simulink model "ScriptDemo"  (R2022b)
settings: configuration reference "TmVcThermal_Configuration_sub" (kept outside this file)
undefined symbols (not defined in the file or in its folder): aaaa, bbbb, cTmComprCtrl_D_u8HvacFlowTable_db, cTmComprCtrl_D_u8HvacFlowTable_sw, cTmComprCtrl_n_i16ChillCmpIMax, cTmComprCtrl_n_i16ChillCmpIMin, cTmComprCtrl_n_i16ChillCmpIMin666, cTmComprCtrl_n_i16ChillCmpPMax, cTmComprCtrl_n_i16ChillCmpPMin, cTmComprCtrl_n_i16CmpChillCoolRpmKiMax, cTmComprCtrl_n_i16CmpChillCoolRpmKiMin, cTmComprCtrl_n_i16CmpChillCoolRpmKpMax, cTmComprCtrl_n_i16CmpChillCoolRpmKpMin, cTmComprCtrl_n_i16CmpCoolRpmKiMax, cTmComprCtrl_n_i16CmpCoolRpmKiMin, cTmComprCtrl_n_i16CmpCoolRpmKpMax, cTmComprCtrl_n_i16CmpCoolRpmKpMin, cTmComprCtrl_n_i16SM4CmpHeatKiMax, cTmComprCtrl_n_i16SM4CmpHeatKiMin, cTmComprCtrl_n_i16SM4CmpHeatKpMax, cTmComprCtrl_n_i16SM4CmpHeatKpMin, cTmComprCtrl_n_i16SM5CmpHeatKiMax, cTmComprCtrl_n_i16SM5CmpHeatKiMin, cTmComprCtrl_n_i16SM5CmpHeatKpMax, cTmComprCtrl_n_i16SM5CmpHeatKpMin, cTmComprCtrl_n_i16SM6CmpHeatKiMax, cTmComprCtrl_n_i16SM6CmpHeatKiMin, cTmComprCtrl_n_i16SM6CmpHeatKpMax, cTmComprCtrl_n_i16SM6CmpHeatKpMin, cTmComprCtrl_n_u16CmpMaxSpdFanFltLimt, cTmComprCtrl_n_u16CmpMaxSpdLoSidePFltLimt, cTmComprCtrl_n_u16CmpMaxSpdSensorFltLimt, cTmComprCtrl_n_u16CompMinRpm, cTmComprCtrl_n_u16CompRpmIncThres, cTmComprCtrl_t_u16BattCooltFFPeriod, cTmComprCtrl_t_u16BattCooltPIPeriod, cTmComprCtrl_t_u16CmpCoolFFPeriod, cTmComprCtrl_t_u16CmpCoolPIPeriod, cTmComprCtrl_t_u16CoolCmpChillFFPeriod, cTmComprCtrl_t_u16CoolCmpChillPIPeriod, cTmComprCtrl_t_u16SM4CmpHeatFFPeriod, cTmComprCtrl_t_u16SM4CmpHeatPIPeriod, cTmComprCtrl_t_u16SM5CmpHeatFFPeriod, cTmComprCtrl_t_u16SM5CmpHeatPIPeriod, cTmComprCtrl_t_u16SM6CmpHeatFFPeriod, cTmComprCtrl_t_u16SM6CmpHeatPIPeriod, cTmComprCtrl_Te_EvapClearInteg, cTmComprCtrl_Te_i16HpReqTempSaturoffset, cTmComprCtrl_Te_i16SatLpReplaceDiff, cTmComprCtrl_Te_i16SM3BatDiffStartEvapDecOffset, cTmComprCtrl_Te_i16SM3EvapLo, cTmComprCtrl_Te_i16SM3TBatDiffEntEvapDecOffset, cTmComprCtrl_Te_i16SM3TBatDiffEntEvapDecOffsetQuit, cTmComprCtrl_Te_s32ErrCmpChillPIContinueCoolH, cTmComprCtrl_Te_s32ErrCmpChillPIContinueCoolL, cTmComprCtrl_Te_s32ErrCmpPIContinueChillH, cTmComprCtrl_Te_s32ErrCmpPIContinueChillL, cTmComprCtrl_Te_s32ErrCmpPIContinueCoolH, cTmComprCtrl_Te_s32ErrCmpPIContinueCoolL, cTmComprCtrl_Te_s32ErrCmpPIContinueHeatH ... (+398)
libraries: simulink x846, PCMULib x711, simulink_need_slupdate x4
(part 47 of 49)

== system ScriptDemo/Create/createMerge/After/SM3SM23/ID26262_SM3FF/SM3SM2FF/Flow2RpmRec1/Subsystem5 ==
  In1 : Inport  OutDataTypeStr=int16
  Abs : Abs  OutDataTypeStr=uint16  SaturateOnIntegerOverflow=off
  Add6 : Sum  Inputs=+-  OutDataTypeStr=int16
  Compare To Constant : simulink/Logic and Bit Operations/Compare To Constant  relop=>=  const=0  OutDataTypeStr=boolean
  Compare To Constant1 : simulink/Logic and Bit Operations/Compare To Constant  relop=<=  const=10  OutDataTypeStr=boolean
  Constant6 : Constant  Value=0  OutDataTypeStr=uint16
  Constant7 : Constant  Value=10  OutDataTypeStr=uint16
  Logical Operator : Logic  AllPortsSameDT=off  OutDataTypeStr=boolean
  Switch : Switch  Criteria=u2 ~= 0  SaturateOnIntegerOverflow=off  InputSameDT=off
  Out1 : Outport
  wires:
  Add6/1 -> Switch/1
  Logical Operator/1 -> Switch/2
  Constant6/1 -> Switch/3
  Abs/1 -> Add6/2, Compare To Constant/1, Compare To Constant1/1
  Constant7/1 -> Add6/1
  Switch/1 -> Out1/1
  Compare To Constant1/1 -> Logical Operator/2
  Compare To Constant/1 -> Logical Operator/1
  In1/1 -> Abs/1

== system ScriptDemo/Create/createMerge/After/SM3SM23/ID26262_SM3FF/SM3SM2FF/Flow2RpmRec1/XCP ==
  md_u8Blw : Inport
  Constant1 : Constant  Value=BlwHeatLevel_db
      settings: AttributesFormatString=%<Value>
  Constant28 : Constant  Value=BlwHeatLevel_sw
      settings: AttributesFormatString=%<Value>
  Switch : Switch  Criteria=u2 ~= 0  SaturateOnIntegerOverflow=off  InputSameDT=off
  Out1 : Outport
  wires:
  md_u8Blw/1 -> Switch/3
  Switch/1 -> Out1/1
  Constant28/1 -> Switch/2
  Constant1/1 -> Switch/1

== system ScriptDemo/Create/createMerge/After/SM3SM23/ID26263_SM3Error/SM3HPErr/isNeedOffset/Timer Running2 ==
  note: CounterRunning
  note: If timer is set to zero, use start/hold/reset-status as output.
      | This is to avoid TimerFinished to be set to true without even the timer has started.
  Start : Inport  OutDataTypeStr=boolean
  Reset : Inport  Port=2  OutDataTypeStr=boolean
  Time : Inport  Port=3  OutDataTypeStr=uint16
  Divide : Product  Inputs=*/  OutDataTypeStr=uint32  RndMeth=Round  SaturateOnIntegerOverflow=on
  IC : Constant  Value=0  OutDataTypeStr=uint32  SampleTime=-1
  Increment : Constant  OutDataTypeStr=uint32  SampleTime=-1
  Logical Operator : Logic  AllPortsSameDT=off  OutDataTypeStr=boolean
  Logical Operator2 : Logic  Operator=OR  AllPortsSameDT=off  OutDataTypeStr=boolean
  Logical Operator3 : Logic  Operator=NOT  AllPortsSameDT=off  OutDataTypeStr=boolean
  Relational Operator : RelationalOperator  OutDataTypeStr=boolean  InputSameDT=off
  Relational Operator1 : RelationalOperator  Operator=>  OutDataTypeStr=boolean  InputSameDT=off
  RunnablePeriod : Constant  Value=cTmSwArch_t_s32SampleTime  OutDataTypeStr=single  SampleTime=-1
  StopCounter : Constant  Value=0  OutDataTypeStr=uint32  SampleTime=-1
  Sum : Sum  OutDataTypeStr=uint32  SaturateOnIntegerOverflow=on
  Switch : Switch  Criteria=u2 ~= 0  InputSameDT=off
  Switch1 : Switch  Criteria=u2 ~= 0  InputSameDT=off
  Unit Delay External IC : simulink_need_slupdate/Unit Delay External IC  tsamp=-1
  Unit Delay Resettable External IC1 : Subsystem  AncestorBlock=|  mask(Unit Delay Resettable External Initial Condition NGCC v1.0){dataType=uint32}
      | CCMLib/Unit Delay
      | Resettable
      | External IC
      mask prompts: dataType "Data type:"
      mask help:
      | NGCC version of the Simulink built-in block with data type control and boolean datatype usage for internal switch condition.
      | -----------------------------------------------------
      | Normally, the output is the signal u delayed by one sample period.
      | When the reset signal R is true, the state and the output are always set equal to the initial condition signal IC.  This reset action is vectorized and supports scalar expansion.
      |
      | Mx-VDev tested: Yes
      mask TypeOptions dataType: uint8 | uint16 | uint32 | single
      mask Display: dpoly(1,[1 0],'z')
  ZeroTicks : Constant  Value=0  OutDataTypeStr=uint32  SampleTime=-1
  false : Constant  Value=false  OutDataTypeStr=boolean  SampleTime=-1
  TimerFinished : Outport  OutDataTypeStr=boolean
  TimerRunning : Outport  Port=2  OutDataTypeStr=boolean
  wires:
  Logical Operator2/1 -> Logical Operator/1
  false/1 -> Unit Delay External IC/2
  Logical Operator/1 -> Switch/2, Unit Delay External IC/1, Switch1/3, TimerRunning/1
  Start/1 -> Logical Operator2/2
  Unit Delay External IC/1 -> Logical Operator2/1
  Unit Delay Resettable External IC1/1(y) -> Relational Operator/1, Sum/1
  Switch/1 -> Sum/2
  Increment/1 -> Switch/1
  StopCounter/1 -> Switch/3
  RunnablePeriod/1 -> Divide/2
  ZeroTicks/1 -> Relational Operator1/2
  Relational Operator1/1 -> Switch1/2
  Relational Operator/1 -> Switch1/1
  Divide/1 -> Relational Operator/2, Relational Operator1/1
  Switch1/1 -> TimerFinished/1
  Logical Operator3/1 -> Logical Operator/2
  Reset/1 -> Logical Operator3/1, Unit Delay Resettable External IC1/3(R)
  Time/1 -> Divide/1
  IC/1 -> Unit Delay Resettable External IC1/2(IC)
  Sum/1 -> Unit Delay Resettable External IC1/1(u)

== system ScriptDemo/Create/createMerge/After/SM3SM23/SM3_Ki/SM2Ki/Flow2Rpm/Subsystem1 ==
  In1 : Inport  OutDataTypeStr=int16
  Abs : Abs  OutDataTypeStr=single  SaturateOnIntegerOverflow=off
  Add6 : Sum  Inputs=+-  OutDataTypeStr=int16
  Compare To Constant : simulink/Logic and Bit Operations/Compare To Constant  relop=>=  const=0  OutDataTypeStr=boolean
  Compare To Constant1 : simulink/Logic and Bit Operations/Compare To Constant  relop=<=  const=10  OutDataTypeStr=boolean
  Constant6 : Constant  Value=0  OutDataTypeStr=uint16
  Constant7 : Constant  Value=10  OutDataTypeStr=uint16
  Logical Operator : Logic  AllPortsSameDT=off  OutDataTypeStr=boolean
  Switch : Switch  Criteria=u2 ~= 0  SaturateOnIntegerOverflow=off  InputSameDT=off
  Out1 : Outport
  wires:
  Add6/1 -> Switch/1
  Logical Operator/1 -> Switch/2
  Constant6/1 -> Switch/3
  Abs/1 -> Add6/2, Compare To Constant/1, Compare To Constant1/1
  Constant7/1 -> Add6/1
  Switch/1 -> Out1/1
  Compare To Constant1/1 -> Logical Operator/2
  Compare To Constant/1 -> Logical Operator/1
  In1/1 -> Abs/1

== system ScriptDemo/Create/createMerge/After/SM3SM23/SM3_Ki/SM2Ki/Flow2Rpm/Subsystem2 ==
  In1 : Inport  OutDataTypeStr=int16
  Abs : Abs  OutDataTypeStr=uint16  SaturateOnIntegerOverflow=off
  Add6 : Sum  Inputs=+-  OutDataTypeStr=int16
  Compare To Constant : simulink/Logic and Bit Operations/Compare To Constant  relop=>=  const=0  OutDataTypeStr=boolean
  Compare To Constant1 : simulink/Logic and Bit Operations/Compare To Constant  relop=<=  const=10  OutDataTypeStr=boolean
  Constant6 : Constant  Value=0  OutDataTypeStr=uint16
  Constant7 : Constant  Value=10  OutDataTypeStr=uint16
  Logical Operator : Logic  AllPortsSameDT=off  OutDataTypeStr=boolean
  Switch : Switch  Criteria=u2 ~= 0  SaturateOnIntegerOverflow=off  InputSameDT=off
  Out1 : Outport
  wires:
  Add6/1 -> Switch/1
  Logical Operator/1 -> Switch/2
  Constant6/1 -> Switch/3
  Abs/1 -> Add6/2, Compare To Constant/1, Compare To Constant1/1
  Constant7/1 -> Add6/1
  Switch/1 -> Out1/1
  Compare To Constant1/1 -> Logical Operator/2
  Compare To Constant/1 -> Logical Operator/1
  In1/1 -> Abs/1

== system ScriptDemo/Create/createMerge/After/SM3SM23/SM3_Ki/SM2Ki/Flow2Rpm/Subsystem3 ==
  In1 : Inport  OutDataTypeStr=int16
  Abs : Abs  OutDataTypeStr=uint16  SaturateOnIntegerOverflow=off
  Add6 : Sum  Inputs=+-  OutDataTypeStr=int16
  Compare To Constant : simulink/Logic and Bit Operations/Compare To Constant  relop=>=  const=0  OutDataTypeStr=boolean
  Compare To Constant1 : simulink/Logic and Bit Operations/Compare To Constant  relop=<=  const=10  OutDataTypeStr=boolean
  Constant6 : Constant  Value=0  OutDataTypeStr=uint16
  Constant7 : Constant  Value=10  OutDataTypeStr=uint16
  Logical Operator : Logic  AllPortsSameDT=off  OutDataTypeStr=boolean
  Switch : Switch  Criteria=u2 ~= 0  SaturateOnIntegerOverflow=off  InputSameDT=off
  Out1 : Outport
  wires:
  Add6/1 -> Switch/1
  Logical Operator/1 -> Switch/2
  Constant6/1 -> Switch/3
  Abs/1 -> Add6/2, Compare To Constant/1, Compare To Constant1/1
  Constant7/1 -> Add6/1
  Switch/1 -> Out1/1
  Compare To Constant1/1 -> Logical Operator/2
  Compare To Constant/1 -> Logical Operator/1
  In1/1 -> Abs/1

== system ScriptDemo/Create/createMerge/After/SM3SM23/SM3_Ki/SM2Ki/Flow2Rpm/Subsystem4 ==
  In1 : Inport  OutDataTypeStr=int16
  Abs : Abs  OutDataTypeStr=uint16  SaturateOnIntegerOverflow=off
  Add6 : Sum  Inputs=+-  OutDataTypeStr=int16
  Compare To Constant : simulink/Logic and Bit Operations/Compare To Constant  relop=>=  const=0  OutDataTypeStr=boolean
  Compare To Constant1 : simulink/Logic and Bit Operations/Compare To Constant  relop=<=  const=10  OutDataTypeStr=boolean
  Constant6 : Constant  Value=0  OutDataTypeStr=uint16
  Constant7 : Constant  Value=10  OutDataTypeStr=uint16
  Logical Operator : Logic  AllPortsSameDT=off  OutDataTypeStr=boolean
  Switch : Switch  Criteria=u2 ~= 0  SaturateOnIntegerOverflow=off  InputSameDT=off
  Out1 : Outport
  wires:
  Add6/1 -> Switch/1
  Logical Operator/1 -> Switch/2
  Constant6/1 -> Switch/3
  Abs/1 -> Add6/2, Compare To Constant/1, Compare To Constant1/1
  Constant7/1 -> Add6/1
  Switch/1 -> Out1/1
  Compare To Constant1/1 -> Logical Operator/2
  Compare To Constant/1 -> Logical Operator/1
  In1/1 -> Abs/1

== system ScriptDemo/Create/createMerge/After/SM3SM23/SM3_Ki/SM2Ki/Flow2Rpm/Subsystem5 ==
  In1 : Inport  OutDataTypeStr=int16
  Abs : Abs  OutDataTypeStr=uint16  SaturateOnIntegerOverflow=off
  Add6 : Sum  Inputs=+-  OutDataTypeStr=int16
  Compare To Constant : simulink/Logic and Bit Operations/Compare To Constant  relop=>=  const=0  OutDataTypeStr=boolean
  Compare To Constant1 : simulink/Logic and Bit Operations/Compare To Constant  relop=<=  const=10  OutDataTypeStr=boolean
  Constant6 : Constant  Value=0  OutDataTypeStr=uint16
  Constant7 : Constant  Value=10  OutDataTypeStr=uint16
  Logical Operator : Logic  AllPortsSameDT=off  OutDataTypeStr=boolean
  Switch : Switch  Criteria=u2 ~= 0  SaturateOnIntegerOverflow=off  InputSameDT=off
  Out1 : Outport
  wires:
  Add6/1 -> Switch/1
  Logical Operator/1 -> Switch/2
  Constant6/1 -> Switch/3
  Abs/1 -> Add6/2, Compare To Constant/1, Compare To Constant1/1
  Constant7/1 -> Add6/1
  Switch/1 -> Out1/1
  Compare To Constant1/1 -> Logical Operator/2
  Compare To Constant/1 -> Logical Operator/1
  In1/1 -> Abs/1

== system ScriptDemo/Create/createMerge/After/SM3SM23/SM3_Ki/SM2Ki/Flow2Rpm/XCP ==
  md_u8Blw : Inport
  Constant1 : Constant  Value=BlwHeatLevel_db
      settings: AttributesFormatString=%<Value>
  Constant28 : Constant  Value=BlwHeatLevel_sw
      settings: AttributesFormatString=%<Value>
  Switch : Switch  Criteria=u2 ~= 0  SaturateOnIntegerOverflow=off  InputSameDT=off
  Out1 : Outport
  wires:
  md_u8Blw/1 -> Switch/3
  Switch/1 -> Out1/1
  Constant28/1 -> Switch/2
  Constant1/1 -> Switch/1

== system ScriptDemo/Create/createMerge/After/SM3SM23/SM3_Ki/SM2Ki/Flow2Rpm1/Subsystem1 ==
  In1 : Inport  OutDataTypeStr=int16
  Abs : Abs  OutDataTypeStr=single  SaturateOnIntegerOverflow=off
  Add6 : Sum  Inputs=+-  OutDataTypeStr=int16
  Compare To Constant : simulink/Logic and Bit Operations/Compare To Constant  relop=>=  const=0  OutDataTypeStr=boolean
  Compare To Constant1 : simulink/Logic and Bit Operations/Compare To Constant  relop=<=  const=10  OutDataTypeStr=boolean
  Constant6 : Constant  Value=0  OutDataTypeStr=uint16
  Constant7 : Constant  Value=10  OutDataTypeStr=uint16
  Logical Operator : Logic  AllPortsSameDT=off  OutDataTypeStr=boolean
  Switch : Switch  Criteria=u2 ~= 0  SaturateOnIntegerOverflow=off  InputSameDT=off
  Out1 : Outport
  wires:
  Add6/1 -> Switch/1
  Logical Operator/1 -> Switch/2
  Constant6/1 -> Switch/3
  Abs/1 -> Add6/2, Compare To Constant/1, Compare To Constant1/1
  Constant7/1 -> Add6/1
  Switch/1 -> Out1/1
  Compare To Constant1/1 -> Logical Operator/2
  Compare To Constant/1 -> Logical Operator/1
  In1/1 -> Abs/1

== system ScriptDemo/Create/createMerge/After/SM3SM23/SM3_Ki/SM2Ki/Flow2Rpm1/Subsystem2 ==
  In1 : Inport  OutDataTypeStr=int16
  Abs : Abs  OutDataTypeStr=uint16  SaturateOnIntegerOverflow=off
  Add6 : Sum  Inputs=+-  OutDataTypeStr=int16
  Compare To Constant : simulink/Logic and Bit Operations/Compare To Constant  relop=>=  const=0  OutDataTypeStr=boolean
  Compare To Constant1 : simulink/Logic and Bit Operations/Compare To Constant  relop=<=  const=10  OutDataTypeStr=boolean
  Constant6 : Constant  Value=0  OutDataTypeStr=uint16
  Constant7 : Constant  Value=10  OutDataTypeStr=uint16
  Logical Operator : Logic  AllPortsSameDT=off  OutDataTypeStr=boolean
  Switch : Switch  Criteria=u2 ~= 0  SaturateOnIntegerOverflow=off  InputSameDT=off
  Out1 : Outport
  wires:
  Add6/1 -> Switch/1
  Logical Operator/1 -> Switch/2
  Constant6/1 -> Switch/3
  Abs/1 -> Add6/2, Compare To Constant/1, Compare To Constant1/1
  Constant7/1 -> Add6/1
  Switch/1 -> Out1/1
  Compare To Constant1/1 -> Logical Operator/2
  Compare To Constant/1 -> Logical Operator/1
  In1/1 -> Abs/1

== system ScriptDemo/Create/createMerge/After/SM3SM23/SM3_Ki/SM2Ki/Flow2Rpm1/Subsystem3 ==
  In1 : Inport  OutDataTypeStr=int16
  Abs : Abs  OutDataTypeStr=uint16  SaturateOnIntegerOverflow=off
  Add6 : Sum  Inputs=+-  OutDataTypeStr=int16
  Compare To Constant : simulink/Logic and Bit Operations/Compare To Constant  relop=>=  const=0  OutDataTypeStr=boolean
  Compare To Constant1 : simulink/Logic and Bit Operations/Compare To Constant  relop=<=  const=10  OutDataTypeStr=boolean
  Constant6 : Constant  Value=0  OutDataTypeStr=uint16
  Constant7 : Constant  Value=10  OutDataTypeStr=uint16
  Logical Operator : Logic  AllPortsSameDT=off  OutDataTypeStr=boolean
  Switch : Switch  Criteria=u2 ~= 0  SaturateOnIntegerOverflow=off  InputSameDT=off
  Out1 : Outport
  wires:
  Add6/1 -> Switch/1
  Logical Operator/1 -> Switch/2
  Constant6/1 -> Switch/3
  Abs/1 -> Add6/2, Compare To Constant/1, Compare To Constant1/1
  Constant7/1 -> Add6/1
  Switch/1 -> Out1/1
  Compare To Constant1/1 -> Logical Operator/2
  Compare To Constant/1 -> Logical Operator/1
  In1/1 -> Abs/1

== system ScriptDemo/Create/createMerge/After/SM3SM23/SM3_Ki/SM2Ki/Flow2Rpm1/Subsystem4 ==
  In1 : Inport  OutDataTypeStr=int16
  Abs : Abs  OutDataTypeStr=uint16  SaturateOnIntegerOverflow=off
  Add6 : Sum  Inputs=+-  OutDataTypeStr=int16
  Compare To Constant : simulink/Logic and Bit Operations/Compare To Constant  relop=>=  const=0  OutDataTypeStr=boolean
  Compare To Constant1 : simulink/Logic and Bit Operations/Compare To Constant  relop=<=  const=10  OutDataTypeStr=boolean
  Constant6 : Constant  Value=0  OutDataTypeStr=uint16
  Constant7 : Constant  Value=10  OutDataTypeStr=uint16
  Logical Operator : Logic  AllPortsSameDT=off  OutDataTypeStr=boolean
  Switch : Switch  Criteria=u2 ~= 0  SaturateOnIntegerOverflow=off  InputSameDT=off
  Out1 : Outport
  wires:
  Add6/1 -> Switch/1
  Logical Operator/1 -> Switch/2
  Constant6/1 -> Switch/3
  Abs/1 -> Add6/2, Compare To Constant/1, Compare To Constant1/1
  Constant7/1 -> Add6/1
  Switch/1 -> Out1/1
  Compare To Constant1/1 -> Logical Operator/2
  Compare To Constant/1 -> Logical Operator/1
  In1/1 -> Abs/1

== system ScriptDemo/Create/createMerge/After/SM3SM23/SM3_Ki/SM2Ki/Flow2Rpm1/Subsystem5 ==
  In1 : Inport  OutDataTypeStr=int16
  Abs : Abs  OutDataTypeStr=uint16  SaturateOnIntegerOverflow=off
  Add6 : Sum  Inputs=+-  OutDataTypeStr=int16
  Compare To Constant : simulink/Logic and Bit Operations/Compare To Constant  relop=>=  const=0  OutDataTypeStr=boolean
  Compare To Constant1 : simulink/Logic and Bit Operations/Compare To Constant  relop=<=  const=10  OutDataTypeStr=boolean
  Constant6 : Constant  Value=0  OutDataTypeStr=uint16
  Constant7 : Constant  Value=10  OutDataTypeStr=uint16
  Logical Operator : Logic  AllPortsSameDT=off  OutDataTypeStr=boolean
  Switch : Switch  Criteria=u2 ~= 0  SaturateOnIntegerOverflow=off  InputSameDT=off
  Out1 : Outport
  wires:
  Add6/1 -> Switch/1
  Logical Operator/1 -> Switch/2
  Constant6/1 -> Switch/3
  Abs/1 -> Add6/2, Compare To Constant/1, Compare To Constant1/1
  Constant7/1 -> Add6/1
  Switch/1 -> Out1/1
  Compare To Constant1/1 -> Logical Operator/2
  Compare To Constant/1 -> Logical Operator/1
  In1/1 -> Abs/1

== system ScriptDemo/Create/createMerge/After/SM3SM23/SM3_Ki/SM2Ki/Flow2Rpm1/XCP ==
  md_u8Blw : Inport
  Constant1 : Constant  Value=BlwHeatLevel_db
      settings: AttributesFormatString=%<Value>
  Constant28 : Constant  Value=BlwHeatLevel_sw
      settings: AttributesFormatString=%<Value>
  Switch : Switch  Criteria=u2 ~= 0  SaturateOnIntegerOverflow=off  InputSameDT=off
  Out1 : Outport
  wires:
  md_u8Blw/1 -> Switch/3
  Switch/1 -> Out1/1
  Constant28/1 -> Switch/2
  Constant1/1 -> Switch/1

== system ScriptDemo/Create/createMerge/After/SM3SM23/SM3_Ki/SM3SM2LikeKi/Osa/Subsystem1 ==
  In1 : Inport  OutDataTypeStr=int16
  Abs : Abs  OutDataTypeStr=single  SaturateOnIntegerOverflow=off
  Add6 : Sum  Inputs=+-  OutDataTypeStr=int16
  Compare To Constant : simulink/Logic and Bit Operations/Compare To Constant  relop=>=  const=0  OutDataTypeStr=boolean
  Compare To Constant1 : simulink/Logic and Bit Operations/Compare To Constant  relop=<=  const=10  OutDataTypeStr=boolean
  Constant6 : Constant  Value=0  OutDataTypeStr=uint16
  Constant7 : Constant  Value=10  OutDataTypeStr=uint16
  Logical Operator : Logic  AllPortsSameDT=off  OutDataTypeStr=boolean
  Switch : Switch  Criteria=u2 ~= 0  SaturateOnIntegerOverflow=off  InputSameDT=off
  Out1 : Outport
  wires:
  Add6/1 -> Switch/1
  Logical Operator/1 -> Switch/2
  Constant6/1 -> Switch/3
  Abs/1 -> Add6/2, Compare To Constant/1, Compare To Constant1/1
  Constant7/1 -> Add6/1
  Switch/1 -> Out1/1
  Compare To Constant1/1 -> Logical Operator/2
  Compare To Constant/1 -> Logical Operator/1
  In1/1 -> Abs/1

== system ScriptDemo/Create/createMerge/After/SM3SM23/SM3_Ki/SM3SM2LikeKi/Osa/Subsystem2 ==
  In1 : Inport  OutDataTypeStr=int16
  Abs : Abs  OutDataTypeStr=uint16  SaturateOnIntegerOverflow=off
  Add6 : Sum  Inputs=+-  OutDataTypeStr=int16
  Compare To Constant : simulink/Logic and Bit Operations/Compare To Constant  relop=>=  const=0  OutDataTypeStr=boolean
  Compare To Constant1 : simulink/Logic and Bit Operations/Compare To Constant  relop=<=  const=10  OutDataTypeStr=boolean
  Constant6 : Constant  Value=0  OutDataTypeStr=uint16
  Constant7 : Constant  Value=10  OutDataTypeStr=uint16
  Logical Operator : Logic  AllPortsSameDT=off  OutDataTypeStr=boolean
  Switch : Switch  Criteria=u2 ~= 0  SaturateOnIntegerOverflow=off  InputSameDT=off
  Out1 : Outport
  wires:
  Add6/1 -> Switch/1
  Logical Operator/1 -> Switch/2
  Constant6/1 -> Switch/3
  Abs/1 -> Add6/2, Compare To Constant/1, Compare To Constant1/1
  Constant7/1 -> Add6/1
  Switch/1 -> Out1/1
  Compare To Constant1/1 -> Logical Operator/2
  Compare To Constant/1 -> Logical Operator/1
  In1/1 -> Abs/1

== system ScriptDemo/Create/createMerge/After/SM3SM23/SM3_Ki/SM3SM2LikeKi/Osa/Subsystem3 ==
  In1 : Inport  OutDataTypeStr=int16
  Abs : Abs  OutDataTypeStr=uint16  SaturateOnIntegerOverflow=off
  Add6 : Sum  Inputs=+-  OutDataTypeStr=int16
  Compare To Constant : simulink/Logic and Bit Operations/Compare To Constant  relop=>=  const=0  OutDataTypeStr=boolean
  Compare To Constant1 : simulink/Logic and Bit Operations/Compare To Constant  relop=<=  const=10  OutDataTypeStr=boolean
  Constant6 : Constant  Value=0  OutDataTypeStr=uint16
  Constant7 : Constant  Value=10  OutDataTypeStr=uint16
  Logical Operator : Logic  AllPortsSameDT=off  OutDataTypeStr=boolean
  Switch : Switch  Criteria=u2 ~= 0  SaturateOnIntegerOverflow=off  InputSameDT=off
  Out1 : Outport
  wires:
  Add6/1 -> Switch/1
  Logical Operator/1 -> Switch/2
  Constant6/1 -> Switch/3
  Abs/1 -> Add6/2, Compare To Constant/1, Compare To Constant1/1
  Constant7/1 -> Add6/1
  Switch/1 -> Out1/1
  Compare To Constant1/1 -> Logical Operator/2
  Compare To Constant/1 -> Logical Operator/1
  In1/1 -> Abs/1

== system ScriptDemo/Create/createMerge/After/SM3SM23/SM3_Ki/SM3SM2LikeKi/Osa/Subsystem4 ==
  In1 : Inport  OutDataTypeStr=int16
  Abs : Abs  OutDataTypeStr=uint16  SaturateOnIntegerOverflow=off
  Add6 : Sum  Inputs=+-  OutDataTypeStr=int16
  Compare To Constant : simulink/Logic and Bit Operations/Compare To Constant  relop=>=  const=0  OutDataTypeStr=boolean
  Compare To Constant1 : simulink/Logic and Bit Operations/Compare To Constant  relop=<=  const=10  OutDataTypeStr=boolean
  Constant6 : Constant  Value=0  OutDataTypeStr=uint16
  Constant7 : Constant  Value=10  OutDataTypeStr=uint16
  Logical Operator : Logic  AllPortsSameDT=off  OutDataTypeStr=boolean
  Switch : Switch  Criteria=u2 ~= 0  SaturateOnIntegerOverflow=off  InputSameDT=off
  Out1 : Outport
  wires:
  Add6/1 -> Switch/1
  Logical Operator/1 -> Switch/2
  Constant6/1 -> Switch/3
  Abs/1 -> Add6/2, Compare To Constant/1, Compare To Constant1/1
  Constant7/1 -> Add6/1
  Switch/1 -> Out1/1
  Compare To Constant1/1 -> Logical Operator/2
  Compare To Constant/1 -> Logical Operator/1
  In1/1 -> Abs/1

== system ScriptDemo/Create/createMerge/After/SM3SM23/SM3_Ki/SM3SM2LikeKi/Osa/Subsystem5 ==
  In1 : Inport  OutDataTypeStr=int16
  Abs : Abs  OutDataTypeStr=uint16  SaturateOnIntegerOverflow=off
  Add6 : Sum  Inputs=+-  OutDataTypeStr=int16
  Compare To Constant : simulink/Logic and Bit Operations/Compare To Constant  relop=>=  const=0  OutDataTypeStr=boolean
  Compare To Constant1 : simulink/Logic and Bit Operations/Compare To Constant  relop=<=  const=10  OutDataTypeStr=boolean
  Constant6 : Constant  Value=0  OutDataTypeStr=uint16
  Constant7 : Constant  Value=10  OutDataTypeStr=uint16
  Logical Operator : Logic  AllPortsSameDT=off  OutDataTypeStr=boolean
  Switch : Switch  Criteria=u2 ~= 0  SaturateOnIntegerOverflow=off  InputSameDT=off
  Out1 : Outport
  wires:
  Add6/1 -> Switch/1
  Logical Operator/1 -> Switch/2
  Constant6/1 -> Switch/3
  Abs/1 -> Add6/2, Compare To Constant/1, Compare To Constant1/1
  Constant7/1 -> Add6/1
  Switch/1 -> Out1/1
  Compare To Constant1/1 -> Logical Operator/2
  Compare To Constant/1 -> Logical Operator/1
  In1/1 -> Abs/1

== system ScriptDemo/Create/createMerge/After/SM3SM23/SM3_Ki/SM3SM2LikeKi/Osa/XCP ==
  md_u8Blw : Inport
  Constant1 : Constant  Value=BlwHeatLevel_db
      settings: AttributesFormatString=%<Value>
  Constant28 : Constant  Value=BlwHeatLevel_sw
      settings: AttributesFormatString=%<Value>
  Switch : Switch  Criteria=u2 ~= 0  SaturateOnIntegerOverflow=off  InputSameDT=off
  Out1 : Outport
  wires:
  md_u8Blw/1 -> Switch/3
  Switch/1 -> Out1/1
  Constant28/1 -> Switch/2
  Constant1/1 -> Switch/1

== system ScriptDemo/Create/createMerge/After/SM3SM23/SM3_Ki/SM3SM2LikeKi/Rec/Subsystem1 ==
  In1 : Inport  OutDataTypeStr=int16
  Abs : Abs  OutDataTypeStr=single  SaturateOnIntegerOverflow=off
  Add6 : Sum  Inputs=+-  OutDataTypeStr=int16
  Compare To Constant : simulink/Logic and Bit Operations/Compare To Constant  relop=>=  const=0  OutDataTypeStr=boolean
  Compare To Constant1 : simulink/Logic and Bit Operations/Compare To Constant  relop=<=  const=10  OutDataTypeStr=boolean
  Constant6 : Constant  Value=0  OutDataTypeStr=uint16
  Constant7 : Constant  Value=10  OutDataTypeStr=uint16
  Logical Operator : Logic  AllPortsSameDT=off  OutDataTypeStr=boolean
  Switch : Switch  Criteria=u2 ~= 0  SaturateOnIntegerOverflow=off  InputSameDT=off
  Out1 : Outport
  wires:
  Add6/1 -> Switch/1
  Logical Operator/1 -> Switch/2
  Constant6/1 -> Switch/3
  Abs/1 -> Add6/2, Compare To Constant/1, Compare To Constant1/1
  Constant7/1 -> Add6/1
  Switch/1 -> Out1/1
  Compare To Constant1/1 -> Logical Operator/2
  Compare To Constant/1 -> Logical Operator/1
  In1/1 -> Abs/1

== system ScriptDemo/Create/createMerge/After/SM3SM23/SM3_Ki/SM3SM2LikeKi/Rec/Subsystem2 ==
  In1 : Inport  OutDataTypeStr=int16
  Abs : Abs  OutDataTypeStr=uint16  SaturateOnIntegerOverflow=off
  Add6 : Sum  Inputs=+-  OutDataTypeStr=int16
  Compare To Constant : simulink/Logic and Bit Operations/Compare To Constant  relop=>=  const=0  OutDataTypeStr=boolean
  Compare To Constant1 : simulink/Logic and Bit Operations/Compare To Constant  relop=<=  const=10  OutDataTypeStr=boolean
  Constant6 : Constant  Value=0  OutDataTypeStr=uint16
  Constant7 : Constant  Value=10  OutDataTypeStr=uint16
  Logical Operator : Logic  AllPortsSameDT=off  OutDataTypeStr=boolean
  Switch : Switch  Criteria=u2 ~= 0  SaturateOnIntegerOverflow=off  InputSameDT=off
  Out1 : Outport
  wires:
  Add6/1 -> Switch/1
  Logical Operator/1 -> Switch/2
  Constant6/1 -> Switch/3
  Abs/1 -> Add6/2, Compare To Constant/1, Compare To Constant1/1
  Constant7/1 -> Add6/1
  Switch/1 -> Out1/1
  Compare To Constant1/1 -> Logical Operator/2
  Compare To Constant/1 -> Logical Operator/1
  In1/1 -> Abs/1

== system ScriptDemo/Create/createMerge/After/SM3SM23/SM3_Ki/SM3SM2LikeKi/Rec/Subsystem3 ==
  In1 : Inport  OutDataTypeStr=int16
  Abs : Abs  OutDataTypeStr=uint16  SaturateOnIntegerOverflow=off
  Add6 : Sum  Inputs=+-  OutDataTypeStr=int16
  Compare To Constant : simulink/Logic and Bit Operations/Compare To Constant  relop=>=  const=0  OutDataTypeStr=boolean
  Compare To Constant1 : simulink/Logic and Bit Operations/Compare To Constant  relop=<=  const=10  OutDataTypeStr=boolean
  Constant6 : Constant  Value=0  OutDataTypeStr=uint16
  Constant7 : Constant  Value=10  OutDataTypeStr=uint16
  Logical Operator : Logic  AllPortsSameDT=off  OutDataTypeStr=boolean
  Switch : Switch  Criteria=u2 ~= 0  SaturateOnIntegerOverflow=off  InputSameDT=off
  Out1 : Outport
  wires:
  Add6/1 -> Switch/1
  Logical Operator/1 -> Switch/2
  Constant6/1 -> Switch/3
  Abs/1 -> Add6/2, Compare To Constant/1, Compare To Constant1/1
  Constant7/1 -> Add6/1
  Switch/1 -> Out1/1
  Compare To Constant1/1 -> Logical Operator/2
  Compare To Constant/1 -> Logical Operator/1
  In1/1 -> Abs/1

== system ScriptDemo/Create/createMerge/After/SM3SM23/SM3_Ki/SM3SM2LikeKi/Rec/Subsystem4 ==
  In1 : Inport  OutDataTypeStr=int16
  Abs : Abs  OutDataTypeStr=uint16  SaturateOnIntegerOverflow=off
  Add6 : Sum  Inputs=+-  OutDataTypeStr=int16
  Compare To Constant : simulink/Logic and Bit Operations/Compare To Constant  relop=>=  const=0  OutDataTypeStr=boolean
  Compare To Constant1 : simulink/Logic and Bit Operations/Compare To Constant  relop=<=  const=10  OutDataTypeStr=boolean
  Constant6 : Constant  Value=0  OutDataTypeStr=uint16
  Constant7 : Constant  Value=10  OutDataTypeStr=uint16
  Logical Operator : Logic  AllPortsSameDT=off  OutDataTypeStr=boolean
  Switch : Switch  Criteria=u2 ~= 0  SaturateOnIntegerOverflow=off  InputSameDT=off
  Out1 : Outport
  wires:
  Add6/1 -> Switch/1
  Logical Operator/1 -> Switch/2
  Constant6/1 -> Switch/3
  Abs/1 -> Add6/2, Compare To Constant/1, Compare To Constant1/1
  Constant7/1 -> Add6/1
  Switch/1 -> Out1/1
  Compare To Constant1/1 -> Logical Operator/2
  Compare To Constant/1 -> Logical Operator/1
  In1/1 -> Abs/1

== system ScriptDemo/Create/createMerge/After/SM3SM23/SM3_Ki/SM3SM2LikeKi/Rec/Subsystem5 ==
  In1 : Inport  OutDataTypeStr=int16
  Abs : Abs  OutDataTypeStr=uint16  SaturateOnIntegerOverflow=off
  Add6 : Sum  Inputs=+-  OutDataTypeStr=int16
  Compare To Constant : simulink/Logic and Bit Operations/Compare To Constant  relop=>=  const=0  OutDataTypeStr=boolean
  Compare To Constant1 : simulink/Logic and Bit Operations/Compare To Constant  relop=<=  const=10  OutDataTypeStr=boolean
  Constant6 : Constant  Value=0  OutDataTypeStr=uint16
  Constant7 : Constant  Value=10  OutDataTypeStr=uint16
  Logical Operator : Logic  AllPortsSameDT=off  OutDataTypeStr=boolean
  Switch : Switch  Criteria=u2 ~= 0  SaturateOnIntegerOverflow=off  InputSameDT=off
  Out1 : Outport
  wires:
  Add6/1 -> Switch/1
  Logical Operator/1 -> Switch/2
  Constant6/1 -> Switch/3
  Abs/1 -> Add6/2, Compare To Constant/1, Compare To Constant1/1
  Constant7/1 -> Add6/1
  Switch/1 -> Out1/1
  Compare To Constant1/1 -> Logical Operator/2
  Compare To Constant/1 -> Logical Operator/1
  In1/1 -> Abs/1

== system ScriptDemo/Create/createMerge/After/SM3SM23/SM3_Ki/SM3SM2LikeKi/Rec/XCP ==
  md_u8Blw : Inport
  Constant1 : Constant  Value=BlwHeatLevel_db
      settings: AttributesFormatString=%<Value>
  Constant28 : Constant  Value=BlwHeatLevel_sw
      settings: AttributesFormatString=%<Value>
  Switch : Switch  Criteria=u2 ~= 0  SaturateOnIntegerOverflow=off  InputSameDT=off
  Out1 : Outport
  wires:
  md_u8Blw/1 -> Switch/3
  Switch/1 -> Out1/1
  Constant28/1 -> Switch/2
  Constant1/1 -> Switch/1

== system ScriptDemo/Create/createMerge/After/SM3SM23/SM3_Kp/SM2Kp/Osa/Subsystem1 ==
  In1 : Inport  OutDataTypeStr=int16
  Abs : Abs  OutDataTypeStr=single  SaturateOnIntegerOverflow=off
  Add6 : Sum  Inputs=+-  OutDataTypeStr=int16
  Compare To Constant : simulink/Logic and Bit Operations/Compare To Constant  relop=>=  const=0  OutDataTypeStr=boolean
  Compare To Constant1 : simulink/Logic and Bit Operations/Compare To Constant  relop=<=  const=10  OutDataTypeStr=boolean
  Constant6 : Constant  Value=0  OutDataTypeStr=uint16
  Constant7 : Constant  Value=10  OutDataTypeStr=uint16
  Logical Operator : Logic  AllPortsSameDT=off  OutDataTypeStr=boolean
  Switch : Switch  Criteria=u2 ~= 0  SaturateOnIntegerOverflow=off  InputSameDT=off
  Out1 : Outport
  wires:
  Add6/1 -> Switch/1
  Logical Operator/1 -> Switch/2
  Constant6/1 -> Switch/3
  Abs/1 -> Add6/2, Compare To Constant/1, Compare To Constant1/1
  Constant7/1 -> Add6/1
  Switch/1 -> Out1/1
  Compare To Constant1/1 -> Logical Operator/2
  Compare To Constant/1 -> Logical Operator/1
  In1/1 -> Abs/1

== system ScriptDemo/Create/createMerge/After/SM3SM23/SM3_Kp/SM2Kp/Osa/Subsystem2 ==
  In1 : Inport  OutDataTypeStr=int16
  Abs : Abs  OutDataTypeStr=uint16  SaturateOnIntegerOverflow=off
  Add6 : Sum  Inputs=+-  OutDataTypeStr=int16
  Compare To Constant : simulink/Logic and Bit Operations/Compare To Constant  relop=>=  const=0  OutDataTypeStr=boolean
  Compare To Constant1 : simulink/Logic and Bit Operations/Compare To Constant  relop=<=  const=10  OutDataTypeStr=boolean
  Constant6 : Constant  Value=0  OutDataTypeStr=uint16
  Constant7 : Constant  Value=10  OutDataTypeStr=uint16
  Logical Operator : Logic  AllPortsSameDT=off  OutDataTypeStr=boolean
  Switch : Switch  Criteria=u2 ~= 0  SaturateOnIntegerOverflow=off  InputSameDT=off
  Out1 : Outport
  wires:
  Add6/1 -> Switch/1
  Logical Operator/1 -> Switch/2
  Constant6/1 -> Switch/3
  Abs/1 -> Add6/2, Compare To Constant/1, Compare To Constant1/1
  Constant7/1 -> Add6/1
  Switch/1 -> Out1/1
  Compare To Constant1/1 -> Logical Operator/2
  Compare To Constant/1 -> Logical Operator/1
  In1/1 -> Abs/1

== system ScriptDemo/Create/createMerge/After/SM3SM23/SM3_Kp/SM2Kp/Osa/Subsystem3 ==
  In1 : Inport  OutDataTypeStr=int16
  Abs : Abs  OutDataTypeStr=uint16  SaturateOnIntegerOverflow=off
  Add6 : Sum  Inputs=+-  OutDataTypeStr=int16
  Compare To Constant : simulink/Logic and Bit Operations/Compare To Constant  relop=>=  const=0  OutDataTypeStr=boolean
  Compare To Constant1 : simulink/Logic and Bit Operations/Compare To Constant  relop=<=  const=10  OutDataTypeStr=boolean
  Constant6 : Constant  Value=0  OutDataTypeStr=uint16
  Constant7 : Constant  Value=10  OutDataTypeStr=uint16
  Logical Operator : Logic  AllPortsSameDT=off  OutDataTypeStr=boolean
  Switch : Switch  Criteria=u2 ~= 0  SaturateOnIntegerOverflow=off  InputSameDT=off
  Out1 : Outport
  wires:
  Add6/1 -> Switch/1
  Logical Operator/1 -> Switch/2
  Constant6/1 -> Switch/3
  Abs/1 -> Add6/2, Compare To Constant/1, Compare To Constant1/1
  Constant7/1 -> Add6/1
  Switch/1 -> Out1/1
  Compare To Constant1/1 -> Logical Operator/2
  Compare To Constant/1 -> Logical Operator/1
  In1/1 -> Abs/1

== system ScriptDemo/Create/createMerge/After/SM3SM23/SM3_Kp/SM2Kp/Osa/Subsystem4 ==
  In1 : Inport  OutDataTypeStr=int16
  Abs : Abs  OutDataTypeStr=uint16  SaturateOnIntegerOverflow=off
  Add6 : Sum  Inputs=+-  OutDataTypeStr=int16
  Compare To Constant : simulink/Logic and Bit Operations/Compare To Constant  relop=>=  const=0  OutDataTypeStr=boolean
  Compare To Constant1 : simulink/Logic and Bit Operations/Compare To Constant  relop=<=  const=10  OutDataTypeStr=boolean
  Constant6 : Constant  Value=0  OutDataTypeStr=uint16
  Constant7 : Constant  Value=10  OutDataTypeStr=uint16
  Logical Operator : Logic  AllPortsSameDT=off  OutDataTypeStr=boolean
  Switch : Switch  Criteria=u2 ~= 0  SaturateOnIntegerOverflow=off  InputSameDT=off
  Out1 : Outport
  wires:
  Add6/1 -> Switch/1
  Logical Operator/1 -> Switch/2
  Constant6/1 -> Switch/3
  Abs/1 -> Add6/2, Compare To Constant/1, Compare To Constant1/1
  Constant7/1 -> Add6/1
  Switch/1 -> Out1/1
  Compare To Constant1/1 -> Logical Operator/2
  Compare To Constant/1 -> Logical Operator/1
  In1/1 -> Abs/1

== system ScriptDemo/Create/createMerge/After/SM3SM23/SM3_Kp/SM2Kp/Osa/Subsystem5 ==
  In1 : Inport  OutDataTypeStr=int16
  Abs : Abs  OutDataTypeStr=uint16  SaturateOnIntegerOverflow=off
  Add6 : Sum  Inputs=+-  OutDataTypeStr=int16
  Compare To Constant : simulink/Logic and Bit Operations/Compare To Constant  relop=>=  const=0  OutDataTypeStr=boolean
  Compare To Constant1 : simulink/Logic and Bit Operations/Compare To Constant  relop=<=  const=10  OutDataTypeStr=boolean
  Constant6 : Constant  Value=0  OutDataTypeStr=uint16
  Constant7 : Constant  Value=10  OutDataTypeStr=uint16
  Logical Operator : Logic  AllPortsSameDT=off  OutDataTypeStr=boolean
  Switch : Switch  Criteria=u2 ~= 0  SaturateOnIntegerOverflow=off  InputSameDT=off
  Out1 : Outport
  wires:
  Add6/1 -> Switch/1
  Logical Operator/1 -> Switch/2
  Constant6/1 -> Switch/3
  Abs/1 -> Add6/2, Compare To Constant/1, Compare To Constant1/1
  Constant7/1 -> Add6/1
  Switch/1 -> Out1/1
  Compare To Constant1/1 -> Logical Operator/2
  Compare To Constant/1 -> Logical Operator/1
  In1/1 -> Abs/1

== system ScriptDemo/Create/createMerge/After/SM3SM23/SM3_Kp/SM2Kp/Osa/XCP ==
  md_u8Blw : Inport
  Constant1 : Constant  Value=BlwHeatLevel_db
      settings: AttributesFormatString=%<Value>
  Constant28 : Constant  Value=BlwHeatLevel_sw
      settings: AttributesFormatString=%<Value>
  Switch : Switch  Criteria=u2 ~= 0  SaturateOnIntegerOverflow=off  InputSameDT=off
  Out1 : Outport
  wires:
  md_u8Blw/1 -> Switch/3
  Switch/1 -> Out1/1
  Constant28/1 -> Switch/2
  Constant1/1 -> Switch/1

== system ScriptDemo/Create/createMerge/After/SM3SM23/SM3_Kp/SM2Kp/Rec/Subsystem1 ==
  In1 : Inport  OutDataTypeStr=int16
  Abs : Abs  OutDataTypeStr=single  SaturateOnIntegerOverflow=off
  Add6 : Sum  Inputs=+-  OutDataTypeStr=int16
  Compare To Constant : simulink/Logic and Bit Operations/Compare To Constant  relop=>=  const=0  OutDataTypeStr=boolean
  Compare To Constant1 : simulink/Logic and Bit Operations/Compare To Constant  relop=<=  const=10  OutDataTypeStr=boolean
  Constant6 : Constant  Value=0  OutDataTypeStr=uint16
  Constant7 : Constant  Value=10  OutDataTypeStr=uint16
  Logical Operator : Logic  AllPortsSameDT=off  OutDataTypeStr=boolean
  Switch : Switch  Criteria=u2 ~= 0  SaturateOnIntegerOverflow=off  InputSameDT=off
  Out1 : Outport
  wires:
  Add6/1 -> Switch/1
  Logical Operator/1 -> Switch/2
  Constant6/1 -> Switch/3
  Abs/1 -> Add6/2, Compare To Constant/1, Compare To Constant1/1
  Constant7/1 -> Add6/1
  Switch/1 -> Out1/1
  Compare To Constant1/1 -> Logical Operator/2
  Compare To Constant/1 -> Logical Operator/1
  In1/1 -> Abs/1

== system ScriptDemo/Create/createMerge/After/SM3SM23/SM3_Kp/SM2Kp/Rec/Subsystem2 ==
  In1 : Inport  OutDataTypeStr=int16
  Abs : Abs  OutDataTypeStr=uint16  SaturateOnIntegerOverflow=off
  Add6 : Sum  Inputs=+-  OutDataTypeStr=int16
  Compare To Constant : simulink/Logic and Bit Operations/Compare To Constant  relop=>=  const=0  OutDataTypeStr=boolean
  Compare To Constant1 : simulink/Logic and Bit Operations/Compare To Constant  relop=<=  const=10  OutDataTypeStr=boolean
  Constant6 : Constant  Value=0  OutDataTypeStr=uint16
  Constant7 : Constant  Value=10  OutDataTypeStr=uint16
  Logical Operator : Logic  AllPortsSameDT=off  OutDataTypeStr=boolean
  Switch : Switch  Criteria=u2 ~= 0  SaturateOnIntegerOverflow=off  InputSameDT=off
  Out1 : Outport
  wires:
  Add6/1 -> Switch/1
  Logical Operator/1 -> Switch/2
  Constant6/1 -> Switch/3
  Abs/1 -> Add6/2, Compare To Constant/1, Compare To Constant1/1
  Constant7/1 -> Add6/1
  Switch/1 -> Out1/1
  Compare To Constant1/1 -> Logical Operator/2
  Compare To Constant/1 -> Logical Operator/1
  In1/1 -> Abs/1

== system ScriptDemo/Create/createMerge/After/SM3SM23/SM3_Kp/SM2Kp/Rec/Subsystem3 ==
  In1 : Inport  OutDataTypeStr=int16
  Abs : Abs  OutDataTypeStr=uint16  SaturateOnIntegerOverflow=off
  Add6 : Sum  Inputs=+-  OutDataTypeStr=int16
  Compare To Constant : simulink/Logic and Bit Operations/Compare To Constant  relop=>=  const=0  OutDataTypeStr=boolean
  Compare To Constant1 : simulink/Logic and Bit Operations/Compare To Constant  relop=<=  const=10  OutDataTypeStr=boolean
  Constant6 : Constant  Value=0  OutDataTypeStr=uint16
  Constant7 : Constant  Value=10  OutDataTypeStr=uint16
  Logical Operator : Logic  AllPortsSameDT=off  OutDataTypeStr=boolean
  Switch : Switch  Criteria=u2 ~= 0  SaturateOnIntegerOverflow=off  InputSameDT=off
  Out1 : Outport
  wires:
  Add6/1 -> Switch/1
  Logical Operator/1 -> Switch/2
  Constant6/1 -> Switch/3
  Abs/1 -> Add6/2, Compare To Constant/1, Compare To Constant1/1
  Constant7/1 -> Add6/1
  Switch/1 -> Out1/1
  Compare To Constant1/1 -> Logical Operator/2
  Compare To Constant/1 -> Logical Operator/1
  In1/1 -> Abs/1

== system ScriptDemo/Create/createMerge/After/SM3SM23/SM3_Kp/SM2Kp/Rec/Subsystem4 ==
  In1 : Inport  OutDataTypeStr=int16
  Abs : Abs  OutDataTypeStr=uint16  SaturateOnIntegerOverflow=off
  Add6 : Sum  Inputs=+-  OutDataTypeStr=int16
  Compare To Constant : simulink/Logic and Bit Operations/Compare To Constant  relop=>=  const=0  OutDataTypeStr=boolean
  Compare To Constant1 : simulink/Logic and Bit Operations/Compare To Constant  relop=<=  const=10  OutDataTypeStr=boolean
  Constant6 : Constant  Value=0  OutDataTypeStr=uint16
  Constant7 : Constant  Value=10  OutDataTypeStr=uint16
  Logical Operator : Logic  AllPortsSameDT=off  OutDataTypeStr=boolean
  Switch : Switch  Criteria=u2 ~= 0  SaturateOnIntegerOverflow=off  InputSameDT=off
  Out1 : Outport
  wires:
  Add6/1 -> Switch/1
  Logical Operator/1 -> Switch/2
  Constant6/1 -> Switch/3
  Abs/1 -> Add6/2, Compare To Constant/1, Compare To Constant1/1
  Constant7/1 -> Add6/1
  Switch/1 -> Out1/1
  Compare To Constant1/1 -> Logical Operator/2
  Compare To Constant/1 -> Logical Operator/1
  In1/1 -> Abs/1

== system ScriptDemo/Create/createMerge/After/SM3SM23/SM3_Kp/SM2Kp/Rec/Subsystem5 ==
  In1 : Inport  OutDataTypeStr=int16
  Abs : Abs  OutDataTypeStr=uint16  SaturateOnIntegerOverflow=off
  Add6 : Sum  Inputs=+-  OutDataTypeStr=int16
  Compare To Constant : simulink/Logic and Bit Operations/Compare To Constant  relop=>=  const=0  OutDataTypeStr=boolean
  Compare To Constant1 : simulink/Logic and Bit Operations/Compare To Constant  relop=<=  const=10  OutDataTypeStr=boolean
  Constant6 : Constant  Value=0  OutDataTypeStr=uint16
  Constant7 : Constant  Value=10  OutDataTypeStr=uint16
  Logical Operator : Logic  AllPortsSameDT=off  OutDataTypeStr=boolean
  Switch : Switch  Criteria=u2 ~= 0  SaturateOnIntegerOverflow=off  InputSameDT=off
  Out1 : Outport
  wires:
  Add6/1 -> Switch/1
  Logical Operator/1 -> Switch/2
  Constant6/1 -> Switch/3
  Abs/1 -> Add6/2, Compare To Constant/1, Compare To Constant1/1
  Constant7/1 -> Add6/1
  Switch/1 -> Out1/1
  Compare To Constant1/1 -> Logical Operator/2
  Compare To Constant/1 -> Logical Operator/1
  In1/1 -> Abs/1

== system ScriptDemo/Create/createMerge/After/SM3SM23/SM3_Kp/SM2Kp/Rec/XCP ==
  md_u8Blw : Inport
  Constant1 : Constant  Value=BlwHeatLevel_db
      settings: AttributesFormatString=%<Value>
  Constant28 : Constant  Value=BlwHeatLevel_sw
      settings: AttributesFormatString=%<Value>
  Switch : Switch  Criteria=u2 ~= 0  SaturateOnIntegerOverflow=off  InputSameDT=off
  Out1 : Outport
  wires:
  md_u8Blw/1 -> Switch/3
  Switch/1 -> Out1/1
  Constant28/1 -> Switch/2
  Constant1/1 -> Switch/1

== system ScriptDemo/Create/createMerge/After/SM3SM23/SM3_Kp/SM3SM2LikeKp/Osa/Subsystem1 ==
  In1 : Inport  OutDataTypeStr=int16
  Abs : Abs  OutDataTypeStr=single  SaturateOnIntegerOverflow=off
  Add6 : Sum  Inputs=+-  OutDataTypeStr=int16
  Compare To Constant : simulink/Logic and Bit Operations/Compare To Constant  relop=>=  const=0  OutDataTypeStr=boolean
  Compare To Constant1 : simulink/Logic and Bit Operations/Compare To Constant  relop=<=  const=10  OutDataTypeStr=boolean
  Constant6 : Constant  Value=0  OutDataTypeStr=uint16
  Constant7 : Constant  Value=10  OutDataTypeStr=uint16
  Logical Operator : Logic  AllPortsSameDT=off  OutDataTypeStr=boolean
  Switch : Switch  Criteria=u2 ~= 0  SaturateOnIntegerOverflow=off  InputSameDT=off
  Out1 : Outport
  wires:
  Add6/1 -> Switch/1
  Logical Operator/1 -> Switch/2
  Constant6/1 -> Switch/3
  Abs/1 -> Add6/2, Compare To Constant/1, Compare To Constant1/1
  Constant7/1 -> Add6/1
  Switch/1 -> Out1/1
  Compare To Constant1/1 -> Logical Operator/2
  Compare To Constant/1 -> Logical Operator/1
  In1/1 -> Abs/1

== system ScriptDemo/Create/createMerge/After/SM3SM23/SM3_Kp/SM3SM2LikeKp/Osa/Subsystem2 ==
  In1 : Inport  OutDataTypeStr=int16
  Abs : Abs  OutDataTypeStr=uint16  SaturateOnIntegerOverflow=off
  Add6 : Sum  Inputs=+-  OutDataTypeStr=int16
  Compare To Constant : simulink/Logic and Bit Operations/Compare To Constant  relop=>=  const=0  OutDataTypeStr=boolean
  Compare To Constant1 : simulink/Logic and Bit Operations/Compare To Constant  relop=<=  const=10  OutDataTypeStr=boolean
  Constant6 : Constant  Value=0  OutDataTypeStr=uint16
  Constant7 : Constant  Value=10  OutDataTypeStr=uint16
  Logical Operator : Logic  AllPortsSameDT=off  OutDataTypeStr=boolean
  Switch : Switch  Criteria=u2 ~= 0  SaturateOnIntegerOverflow=off  InputSameDT=off
  Out1 : Outport
  wires:
  Add6/1 -> Switch/1
  Logical Operator/1 -> Switch/2
  Constant6/1 -> Switch/3
  Abs/1 -> Add6/2, Compare To Constant/1, Compare To Constant1/1
  Constant7/1 -> Add6/1
  Switch/1 -> Out1/1
  Compare To Constant1/1 -> Logical Operator/2
  Compare To Constant/1 -> Logical Operator/1
  In1/1 -> Abs/1

== system ScriptDemo/Create/createMerge/After/SM3SM23/SM3_Kp/SM3SM2LikeKp/Osa/Subsystem3 ==
  In1 : Inport  OutDataTypeStr=int16
  Abs : Abs  OutDataTypeStr=uint16  SaturateOnIntegerOverflow=off
  Add6 : Sum  Inputs=+-  OutDataTypeStr=int16
  Compare To Constant : simulink/Logic and Bit Operations/Compare To Constant  relop=>=  const=0  OutDataTypeStr=boolean
  Compare To Constant1 : simulink/Logic and Bit Operations/Compare To Constant  relop=<=  const=10  OutDataTypeStr=boolean
  Constant6 : Constant  Value=0  OutDataTypeStr=uint16
  Constant7 : Constant  Value=10  OutDataTypeStr=uint16
  Logical Operator : Logic  AllPortsSameDT=off  OutDataTypeStr=boolean
  Switch : Switch  Criteria=u2 ~= 0  SaturateOnIntegerOverflow=off  InputSameDT=off
  Out1 : Outport
  wires:
  Add6/1 -> Switch/1
  Logical Operator/1 -> Switch/2
  Constant6/1 -> Switch/3
  Abs/1 -> Add6/2, Compare To Constant/1, Compare To Constant1/1
  Constant7/1 -> Add6/1
  Switch/1 -> Out1/1
  Compare To Constant1/1 -> Logical Operator/2
  Compare To Constant/1 -> Logical Operator/1
  In1/1 -> Abs/1

== system ScriptDemo/Create/createMerge/After/SM3SM23/SM3_Kp/SM3SM2LikeKp/Osa/Subsystem4 ==
  In1 : Inport  OutDataTypeStr=int16
  Abs : Abs  OutDataTypeStr=uint16  SaturateOnIntegerOverflow=off
  Add6 : Sum  Inputs=+-  OutDataTypeStr=int16
  Compare To Constant : simulink/Logic and Bit Operations/Compare To Constant  relop=>=  const=0  OutDataTypeStr=boolean
  Compare To Constant1 : simulink/Logic and Bit Operations/Compare To Constant  relop=<=  const=10  OutDataTypeStr=boolean
  Constant6 : Constant  Value=0  OutDataTypeStr=uint16
  Constant7 : Constant  Value=10  OutDataTypeStr=uint16
  Logical Operator : Logic  AllPortsSameDT=off  OutDataTypeStr=boolean
  Switch : Switch  Criteria=u2 ~= 0  SaturateOnIntegerOverflow=off  InputSameDT=off
  Out1 : Outport
  wires:
  Add6/1 -> Switch/1
  Logical Operator/1 -> Switch/2
  Constant6/1 -> Switch/3
  Abs/1 -> Add6/2, Compare To Constant/1, Compare To Constant1/1
  Constant7/1 -> Add6/1
  Switch/1 -> Out1/1
  Compare To Constant1/1 -> Logical Operator/2
  Compare To Constant/1 -> Logical Operator/1
  In1/1 -> Abs/1

== system ScriptDemo/Create/createMerge/After/SM3SM23/SM3_Kp/SM3SM2LikeKp/Osa/Subsystem5 ==
  In1 : Inport  OutDataTypeStr=int16
  Abs : Abs  OutDataTypeStr=uint16  SaturateOnIntegerOverflow=off
  Add6 : Sum  Inputs=+-  OutDataTypeStr=int16
  Compare To Constant : simulink/Logic and Bit Operations/Compare To Constant  relop=>=  const=0  OutDataTypeStr=boolean
  Compare To Constant1 : simulink/Logic and Bit Operations/Compare To Constant  relop=<=  const=10  OutDataTypeStr=boolean
  Constant6 : Constant  Value=0  OutDataTypeStr=uint16
  Constant7 : Constant  Value=10  OutDataTypeStr=uint16
  Logical Operator : Logic  AllPortsSameDT=off  OutDataTypeStr=boolean
  Switch : Switch  Criteria=u2 ~= 0  SaturateOnIntegerOverflow=off  InputSameDT=off
  Out1 : Outport
  wires:
  Add6/1 -> Switch/1
  Logical Operator/1 -> Switch/2
  Constant6/1 -> Switch/3
  Abs/1 -> Add6/2, Compare To Constant/1, Compare To Constant1/1
  Constant7/1 -> Add6/1
  Switch/1 -> Out1/1
  Compare To Constant1/1 -> Logical Operator/2
  Compare To Constant/1 -> Logical Operator/1
  In1/1 -> Abs/1

== system ScriptDemo/Create/createMerge/After/SM3SM23/SM3_Kp/SM3SM2LikeKp/Osa/XCP ==
  md_u8Blw : Inport
  Constant1 : Constant  Value=BlwHeatLevel_db
      settings: AttributesFormatString=%<Value>
  Constant28 : Constant  Value=BlwHeatLevel_sw
      settings: AttributesFormatString=%<Value>
  Switch : Switch  Criteria=u2 ~= 0  SaturateOnIntegerOverflow=off  InputSameDT=off
  Out1 : Outport
  wires:
  md_u8Blw/1 -> Switch/3
  Switch/1 -> Out1/1
  Constant28/1 -> Switch/2
  Constant1/1 -> Switch/1

== system ScriptDemo/Create/createMerge/After/SM3SM23/SM3_Kp/SM3SM2LikeKp/Rec/Subsystem1 ==
  In1 : Inport  OutDataTypeStr=int16
  Abs : Abs  OutDataTypeStr=single  SaturateOnIntegerOverflow=off
  Add6 : Sum  Inputs=+-  OutDataTypeStr=int16
  Compare To Constant : simulink/Logic and Bit Operations/Compare To Constant  relop=>=  const=0  OutDataTypeStr=boolean
  Compare To Constant1 : simulink/Logic and Bit Operations/Compare To Constant  relop=<=  const=10  OutDataTypeStr=boolean
  Constant6 : Constant  Value=0  OutDataTypeStr=uint16
  Constant7 : Constant  Value=10  OutDataTypeStr=uint16
  Logical Operator : Logic  AllPortsSameDT=off  OutDataTypeStr=boolean
  Switch : Switch  Criteria=u2 ~= 0  SaturateOnIntegerOverflow=off  InputSameDT=off
  Out1 : Outport
  wires:
  Add6/1 -> Switch/1
  Logical Operator/1 -> Switch/2
  Constant6/1 -> Switch/3
  Abs/1 -> Add6/2, Compare To Constant/1, Compare To Constant1/1
  Constant7/1 -> Add6/1
  Switch/1 -> Out1/1
  Compare To Constant1/1 -> Logical Operator/2
  Compare To Constant/1 -> Logical Operator/1
  In1/1 -> Abs/1
